simulink model "HM_model"  (R2019b)
settings: Solver=VariableStepAuto  StartTime=0.0  StopTime=100.0  RelTol=1e-3
settings Model: Creator=ryanc  LastModifiedBy=ryanc

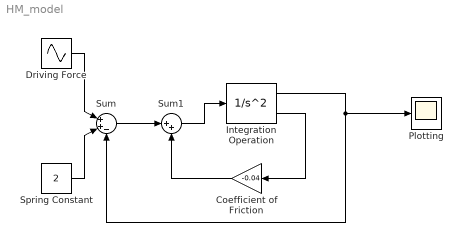
== system HM_model ==
  Coefficient of Friction : Gain  Gain=-0.04
  Driving Force : Sin  Amplitude=0  SampleTime=0
  "Integration Operation " : SecondOrderIntegrator  ICDXDT=2
  "Plotting " : Scope
  Spring Constant : Constant  Value=2
  Sum : Sum  Inputs=|++-
  Sum1 : Sum  Inputs=|++
  wires:
  Spring Constant/1 -> Sum/2
  "Integration Operation "/1 -> Sum/3, "Plotting "/1
  Sum/1 -> Sum1/1
  Sum1/1 -> "Integration Operation "/1
  "Integration Operation "/2 -> Coefficient of Friction/1
  Coefficient of Friction/1 -> Sum1/2
  Driving Force/1 -> Sum/1
